simulink model "UAV_Model_LQR"  (R2018a)
settings: Solver=ode45  StartTime=0.0  StopTime=10  RelTol=1e-3  EnableMultiTasking=on
PreLoadFcn:
  | Imported_Data_old
model workspace: external: MAT-File (data not in the file)
values from neighbouring files (symbols this model uses):
  a1 = (Iyy-Izz)/Ixx    (= -0.733333333333)    [Imported_Data.m]
  a2 = Jr/Ixx    (= 0.008)    [Imported_Data.m]
  a3 = (Izz-Ixx)/Iyy    (= 0.733333333333)    [Imported_Data.m]
  a4 = Jr/Iyy    (= 0.008)    [Imported_Data.m]
  a5 = (Ixx-Iyy)/Izz    (= 0)    [Imported_Data.m]
  b1 = l/Ixx    (= 30.6666666667)    [Imported_Data.m]
  b2 = l/Iyy    (= 30.6666666667)    [Imported_Data.m]
  b3 = 1/Izz    (= 76.9230769231)    [Imported_Data.m]
  g = 9.81    [Imported_Data.m]
  K_hover = [5.69569249622213e-13,1.89531365870451e-15,-1.57466857817560e-15,6.95185031132290e-16,8.39284795530529e-14,4.51806830265205e-16,-17.9474107643174,-11.1054776571569,-7.77632326230154e-14,1.88786479489746e-14,2.53644214862947e-13,1.72488798264706e-13;49.1675228808413,10.1590638141113,-1.10370107195727e-12,-7.50360856396961e-15,-3.02757110244610e-14,-5.68697422933292e-16,-1.57487669583132e-15,-3.7779 ...(+585 chars)    [Imported_Data.m]
  K_i = [-9.99999999999991,-5.72733003083861e-14,1.19859349350458e-13;-1.97870657968378e-15,1.52556519389084e-13,7.07106781186449;1.77273448082462e-14,-7.07106781186519,-4.93357134417905e-13;1.93679622698126e-14,-2.41180621006677e-14,-9.68167127074097e-14]    [Imported_Data.m]
  Kf = 3.13e-5    (= 3.13e-05)    [Imported_Data.m]
  KM = 7.5e-7    (= 7.5e-07)    [Imported_Data.m]
  m = 0.650    (= 0.65)    [Imported_Data.m]
  omega_max = (90/100)*9000*(2*pi/(60))    (= 848.230016469)    [Imported_Data.m]
libraries: simulink_extras x3
settings Model: Creator=ahmad  LastModifiedBy=Ahmad
settings DataIOCC: LimitDataPoints=on  SaveFormat=Array
settings OptimizationCC: LifeSpan=inf
settings DebuggingCC: UnderspecifiedInitializationDetection=Classic  MergeDetectMultiDrivingBlocksExec=none  SolverPrmCheckMsg=warning  StateNameClashWarn=warning  SFUnexpectedBacktrackingDiag=warning  SFNoUnconditionalDefaultTransitionDiag=warning  SFExecutionAtInitializationDiag=none
settings HardwareCC: ProdBitPerPointer=32  ProdBitPerSizeT=32  ProdBitPerPtrDiffT=32  ProdLargestAtomicFloat=None  ProdIntDivRoundTo=Undefined  ProdEndianess=Unspecified  ProdWordSize=32  ProdHWDeviceType=32-bit Generic
settings ModelReferenceCC: PropagateSignalLabelsOutOfModel=off
settings CodeAppCC: StateflowObjectComments=on
settings GRTTargetCC: TargetLangStandard=C89/C90 (ANSI)  GeneratePreprocessorConditionals=Disable all
settings ConfigComp: CovMetricSettings=dw  CovHtmlReporting=on  CovSaveCumulativeToWorkspaceVar=on  CovSaveSingleToWorkspaceVar=on  CovExternalEMLEnable=off
settings SimscapeCC: SimscapeNormalizeSystem=off
settings ConfigurationSet: Description=SimMechanics 2G

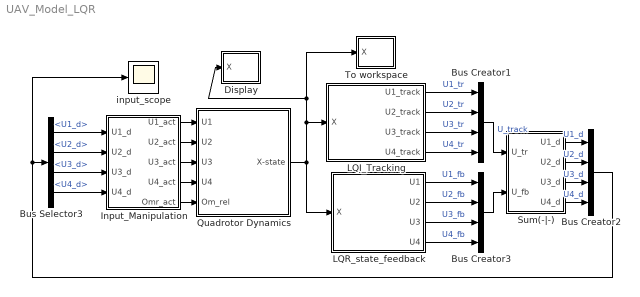
== system UAV_Model_LQR ==
  Bus Creator1 : BusCreator  Inputs=4
  Bus Creator2 : BusCreator  Inputs=4
  Bus Creator3 : BusCreator  Inputs=4
  Bus Selector3 : BusSelector  OutputSignals=U1_d,U2_d,U3_d,U4_d
  Display : Subsystem
  Input_Manipulation : Subsystem
  LQI_Tracking : Subsystem
  LQR_state_feedback : Subsystem
  Quadrotor Dynamics : Subsystem
  Sum(-|-) : Subsystem
  To workspace : Subsystem
  input_scope : Scope
  wires:
  Quadrotor Dynamics/1(X-state) -> LQR_state_feedback/1(X), To workspace/1(X), Display/1(X), LQI_Tracking/1(X)
  LQR_state_feedback/1(U1) -> Bus Creator3/1  "U1_fb"
  LQR_state_feedback/2(U2) -> Bus Creator3/2  "U2_fb"
  LQR_state_feedback/3(U3) -> Bus Creator3/3  "U3_fb"
  LQR_state_feedback/4(U4) -> Bus Creator3/4  "U4_fb"
  Bus Creator3/1 -> Sum(-|-)/2(U_fb)
  Bus Creator2/1 -> input_scope/1, Bus Selector3/1
  Sum(-|-)/1(U1_d) -> Bus Creator2/1  "U1_d"
  Sum(-|-)/2(U2_d) -> Bus Creator2/2  "U2_d"
  Sum(-|-)/3(U3_d) -> Bus Creator2/3  "U3_d"
  Sum(-|-)/4(U4_d) -> Bus Creator2/4  "U4_d"
  LQI_Tracking/1(U1_track) -> Bus Creator1/1  "U1_tr"
  LQI_Tracking/2(U2_track) -> Bus Creator1/2  "U2_tr"
  LQI_Tracking/3(U3_track) -> Bus Creator1/3  "U3_tr"
  Bus Creator1/1 -> Sum(-|-)/1(U_tr)  "U_track"
  LQI_Tracking/4(U4_track) -> Bus Creator1/4  "U4_tr"
  Bus Selector3/1 -> Input_Manipulation/1(U1_d)  "<U1_d>"
  Bus Selector3/2 -> Input_Manipulation/2(U2_d)  "<U2_d>"
  Bus Selector3/3 -> Input_Manipulation/3(U3_d)  "<U3_d>"
  Bus Selector3/4 -> Input_Manipulation/4(U4_d)  "<U4_d>"
  Input_Manipulation/1(U1_act) -> Quadrotor Dynamics/1(U1)
  Input_Manipulation/2(U2_act) -> Quadrotor Dynamics/2(U2)
  Input_Manipulation/3(U3_act) -> Quadrotor Dynamics/3(U3)
  Input_Manipulation/4(U4_act) -> Quadrotor Dynamics/4(U4)
  Input_Manipulation/5(Omr_act) -> Quadrotor Dynamics/5(Om_rel)

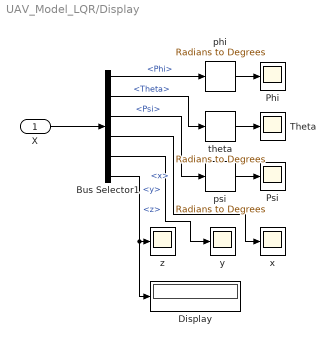
== system UAV_Model_LQR/Display ==
  X : Inport
  Bus Selector1 : BusSelector  OutputSignals=Phi,Theta,Psi,x,y,z
  Display : Display
  Phi : Scope
  Psi : Scope
  "Theta " : Scope
  "phi " : simulink_extras/Transformations/Radians to Degrees
  "psi " : simulink_extras/Transformations/Radians to Degrees
  "theta " : simulink_extras/Transformations/Radians to Degrees
  x : Scope
  y : Scope
  z : Scope
  wires:
  X/1 -> Bus Selector1/1
  Bus Selector1/1 -> "phi "/1  "<Phi>"
  Bus Selector1/2 -> "theta "/1  "<Theta>"
  "theta "/1 -> "Theta "/1
  Bus Selector1/6 -> Display/1, z/1  "<z>"
  Bus Selector1/5 -> y/1  "<y>"
  Bus Selector1/4 -> x/1  "<x>"
  "psi "/1 -> Psi/1
  Bus Selector1/3 -> "psi "/1  "<Psi>"
  "phi "/1 -> Phi/1

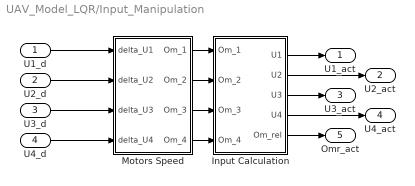
== system UAV_Model_LQR/Input_Manipulation ==
  U1_d : Inport
  U2_d : Inport  Port=2
  U3_d : Inport  Port=3
  U4_d : Inport  Port=4
  Input Calculation : Subsystem
  Motors Speed : Subsystem
  U1_act : Outport
  U2_act : Outport  Port=2
  U3_act : Outport  Port=3
  U4_act : Outport  Port=4
  Omr_act : Outport  Port=5
  wires:
  Input Calculation/1(U1) -> U1_act/1
  Input Calculation/2(U2) -> U2_act/1
  Input Calculation/3(U3) -> U3_act/1
  Input Calculation/4(U4) -> U4_act/1
  Input Calculation/5(Om_rel) -> Omr_act/1
  Motors Speed/1(Om_1) -> Input Calculation/1(Om_1)
  Motors Speed/2(Om_2) -> Input Calculation/2(Om_2)
  Motors Speed/3(Om_3) -> Input Calculation/3(Om_3)
  Motors Speed/4(Om_4) -> Input Calculation/4(Om_4)
  U1_d/1 -> Motors Speed/1(delta_U1)
  U2_d/1 -> Motors Speed/2(delta_U2)
  U3_d/1 -> Motors Speed/3(delta_U3)
  U4_d/1 -> Motors Speed/4(delta_U4)

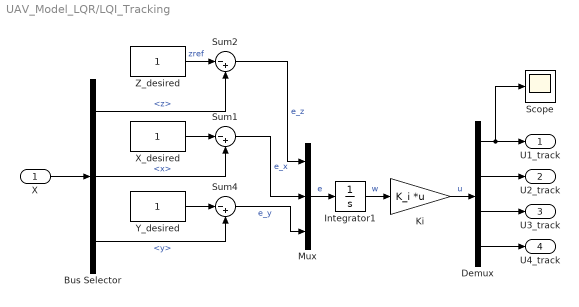
== system UAV_Model_LQR/LQI_Tracking ==
  X : Inport
  Bus Selector : BusSelector  OutputSignals=z,x,y
  Demux : Demux
  Integrator1 : Integrator
  Ki : Gain  Gain=K_i  Multiplication=Matrix(K*u)
  Mux : Mux  Inputs=3
  Scope : Scope
  Sum1 : Sum  Inputs=|-+
  Sum2 : Sum  Inputs=|-+
  Sum4 : Sum  Inputs=|-+
  X_desired : Constant
  Y_desired : Constant
  Z_desired : Constant
  U1_track : Outport
  U2_track : Outport  Port=2
  U3_track : Outport  Port=3
  U4_track : Outport  Port=4
  wires:
  X/1 -> Bus Selector/1
  Demux/1 -> Scope/1, U1_track/1
  Demux/2 -> U2_track/1
  Demux/3 -> U3_track/1
  Demux/4 -> U4_track/1
  Z_desired/1 -> Sum2/1  "zref"
  Ki/1 -> Demux/1  "u"
  Bus Selector/1 -> Sum2/2  "<z>"
  X_desired/1 -> Sum1/1
  Y_desired/1 -> Sum4/1
  Sum1/1 -> Mux/2  "e_x"
  Sum4/1 -> Mux/3  "e_y"
  Sum2/1 -> Mux/1  "e_z"
  Mux/1 -> Integrator1/1  "e"
  Integrator1/1 -> Ki/1  "w"
  Bus Selector/2 -> Sum1/2  "<x>"
  Bus Selector/3 -> Sum4/2  "<y>"

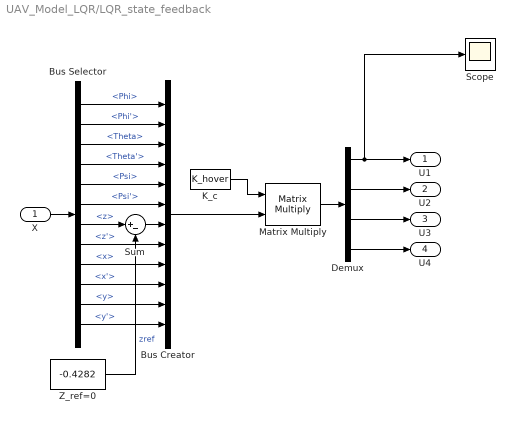
== system UAV_Model_LQR/LQR_state_feedback ==
  X : Inport
  Bus Creator : BusCreator  Inputs=12
  Bus Selector : BusSelector  OutputSignals=Phi,Phi',Theta,Theta',Psi,Psi',z,z',x,x',y,y'
  Demux : Demux
  K_c : Constant  Value=K_hover
  Matrix Multiply : Product  Multiplication=Matrix(*)
  Scope : Scope
  Sum : Sum  Inputs=|+-
  Z_ref=0 : Constant  Value=-0.4282
  U1 : Outport
  U2 : Outport  Port=2
  U3 : Outport  Port=3
  U4 : Outport  Port=4
  wires:
  X/1 -> Bus Selector/1
  Bus Selector/1 -> Bus Creator/1  "<Phi>"
  Bus Selector/2 -> Bus Creator/2  "<Phi'>"
  Bus Selector/3 -> Bus Creator/3  "<Theta>"
  Bus Selector/4 -> Bus Creator/4  "<Theta'>"
  Bus Creator/1 -> Matrix Multiply/2
  K_c/1 -> Matrix Multiply/1
  Bus Selector/7 -> Sum/1  "<z>"
  Bus Selector/8 -> Bus Creator/8  "<z'>"
  Bus Selector/9 -> Bus Creator/9  "<x>"
  Bus Selector/10 -> Bus Creator/10  "<x'>"
  Bus Selector/11 -> Bus Creator/11  "<y>"
  Bus Selector/12 -> Bus Creator/12  "<y'>"
  Z_ref=0/1 -> Sum/2  "zref"
  Sum/1 -> Bus Creator/7
  Demux/1 -> U1/1, Scope/1
  Matrix Multiply/1 -> Demux/1
  Bus Selector/5 -> Bus Creator/5  "<Psi>"
  Bus Selector/6 -> Bus Creator/6  "<Psi'>"
  Demux/2 -> U2/1
  Demux/3 -> U3/1
  Demux/4 -> U4/1

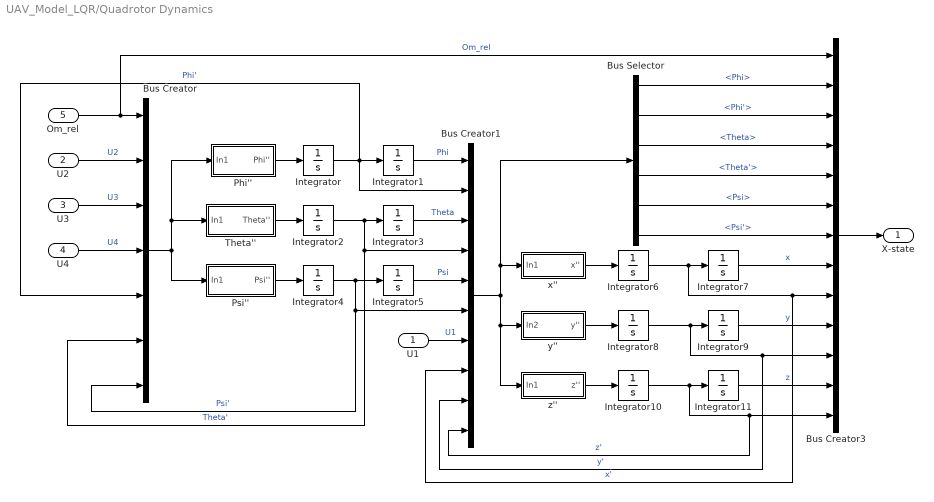
== system UAV_Model_LQR/Quadrotor Dynamics ==
  U1 : Inport
  U2 : Inport  Port=2
  U3 : Inport  Port=3
  U4 : Inport  Port=4
  Om_rel : Inport  Port=5
  Bus Creator : BusCreator  Inputs=7
  Bus Creator1 : BusCreator  Inputs=10
  Bus Creator3 : BusCreator  Inputs=13
  Bus Selector : BusSelector  OutputSignals=Phi,Phi',Theta,Theta',Psi,Psi'
  Integrator{,1..11} (12 alike) : Integrator
  Phi'' : Subsystem
  Psi'' : Subsystem
  Theta'' : Subsystem
  x'' : Subsystem
  y'' : Subsystem
  z'' : Subsystem
  X-state : Outport
  wires:
  Bus Creator/1 -> Phi''/1(In1), Theta''/1(In1), Psi''/1(In1)
  Theta''/1(Theta'') -> Integrator2/1
  Phi''/1(Phi'') -> Integrator/1
  Psi''/1(Psi'') -> Integrator4/1
  Integrator4/1 -> Bus Creator/7, Bus Creator1/6, Integrator5/1  "Psi'"
  Integrator2/1 -> Bus Creator/6, Bus Creator1/4, Integrator3/1  "Theta'"
  Integrator/1 -> Bus Creator1/2, Integrator1/1, Bus Creator/5  "Phi'"
  Om_rel/1 -> Bus Creator3/1, Bus Creator/1  "Om_rel"
  U2/1 -> Bus Creator/2  "U2"
  U3/1 -> Bus Creator/3  "U3"
  U4/1 -> Bus Creator/4  "U4"
  Integrator1/1 -> Bus Creator1/1  "Phi"
  Integrator3/1 -> Bus Creator1/3  "Theta"
  Integrator5/1 -> Bus Creator1/5  "Psi"
  x''/1(x'') -> Integrator6/1
  Integrator6/1 -> Bus Creator3/9, Bus Creator1/8, Integrator7/1  "x'"
  Integrator8/1 -> Integrator9/1, Bus Creator3/11, Bus Creator1/9  "y'"
  Integrator10/1 -> Integrator11/1, Bus Creator3/13, Bus Creator1/10  "z'"
  y''/1(y'') -> Integrator8/1
  z''/1(z'') -> Integrator10/1
  Bus Selector/1 -> Bus Creator3/2  "<Phi>"
  Bus Selector/2 -> Bus Creator3/3  "<Phi'>"
  Bus Selector/3 -> Bus Creator3/4  "<Theta>"
  Bus Selector/4 -> Bus Creator3/5  "<Theta'>"
  Bus Selector/5 -> Bus Creator3/6  "<Psi>"
  Bus Selector/6 -> Bus Creator3/7  "<Psi'>"
  Bus Creator1/1 -> z''/1(In1), y''/1(In2), Bus Selector/1, x''/1(In1)
  Integrator7/1 -> Bus Creator3/8  "x"
  Integrator9/1 -> Bus Creator3/10  "y"
  Integrator11/1 -> Bus Creator3/12  "z"
  U1/1 -> Bus Creator1/7  "U1"
  Bus Creator3/1 -> X-state/1

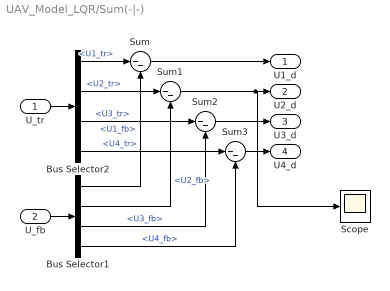
== system UAV_Model_LQR/Sum(-|-) ==
  U_tr : Inport
  U_fb : Inport  Port=2
  Bus Selector1 : BusSelector  OutputSignals=U1_fb,U2_fb,U3_fb,U4_fb
  Bus Selector2 : BusSelector  OutputSignals=U1_tr,U2_tr,U3_tr,U4_tr
  Scope : Scope
  Sum{,1..3} (4 alike) : Sum  Inputs=|--
  U1_d : Outport
  U2_d : Outport  Port=2
  U3_d : Outport  Port=3
  U4_d : Outport  Port=4
  wires:
  U_fb/1 -> Bus Selector1/1
  Bus Selector1/1 -> Sum/2  "<U1_fb>"
  Bus Selector1/2 -> Sum1/2  "<U2_fb>"
  Bus Selector1/3 -> Sum2/2  "<U3_fb>"
  Bus Selector1/4 -> Sum3/2  "<U4_fb>"
  Sum/1 -> U1_d/1
  Sum1/1 -> Scope/1, U2_d/1
  Sum2/1 -> U3_d/1
  Sum3/1 -> U4_d/1
  Bus Selector2/3 -> Sum2/1  "<U3_tr>"
  U_tr/1 -> Bus Selector2/1
  Bus Selector2/1 -> Sum/1  "<U1_tr>"
  Bus Selector2/2 -> Sum1/1  "<U2_tr>"
  Bus Selector2/4 -> Sum3/1  "<U4_tr>"

== system UAV_Model_LQR/To workspace ==
  X : Inport
  Bus Selector2 : BusSelector  OutputSignals=Phi,Theta,Psi,z,y,x
  phi_out : ToWorkspace  VariableName=Phi_out  SaveFormat=Timeseries  SampleTime=-1
  psi_out : ToWorkspace  VariableName=Psi_out  SaveFormat=Timeseries  SampleTime=-1
  theta_out : ToWorkspace  VariableName=Theta_out  SaveFormat=Timeseries  SampleTime=-1
  x_out : ToWorkspace  VariableName=x_out  SaveFormat=Timeseries  SampleTime=-1
  y_out : ToWorkspace  VariableName=y_out  SaveFormat=Timeseries  SampleTime=-1
  z_out : ToWorkspace  VariableName=z_out  SaveFormat=Timeseries  SampleTime=-1
  wires:
  Bus Selector2/1 -> phi_out/1  "<Phi>"
  Bus Selector2/2 -> theta_out/1  "<Theta>"
  Bus Selector2/3 -> psi_out/1  "<Psi>"
  Bus Selector2/4 -> z_out/1  "<z>"
  X/1 -> Bus Selector2/1
  Bus Selector2/5 -> y_out/1  "<y>"
  Bus Selector2/6 -> x_out/1  "<x>"

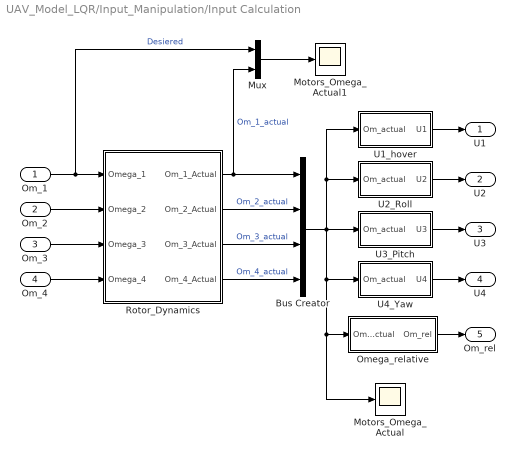
== system UAV_Model_LQR/Input_Manipulation/Input Calculation ==
  Om_1 : Inport
  Om_2 : Inport  Port=2
  Om_3 : Inport  Port=3
  Om_4 : Inport  Port=4
  Bus Creator : BusCreator  Inputs=4
  Motors_Omega_Actual : Scope
  Motors_Omega_Actual1 : Scope
  Mux : Mux  Inputs=2
  Omega_relative : Subsystem
  Rotor_Dynamics : Subsystem
  U1_hover : Subsystem
  U2_Roll : Subsystem
  U3_Pitch : Subsystem
  U4_Yaw : Subsystem
  U1 : Outport
  U2 : Outport  Port=2
  U3 : Outport  Port=3
  U4 : Outport  Port=4
  Om_rel : Outport  Port=5
  wires:
  Om_1/1 -> Mux/1, Rotor_Dynamics/1(Omega_1)  "Desiered"
  Om_3/1 -> Rotor_Dynamics/3(Omega_3)
  Om_2/1 -> Rotor_Dynamics/2(Omega_2)
  Om_4/1 -> Rotor_Dynamics/4(Omega_4)
  Rotor_Dynamics/1(Om_1_Actual) -> Mux/2, Bus Creator/1  "Om_1_actual"
  Rotor_Dynamics/2(Om_2_Actual) -> Bus Creator/2  "Om_2_actual"
  Rotor_Dynamics/3(Om_3_Actual) -> Bus Creator/3  "Om_3_actual"
  Rotor_Dynamics/4(Om_4_Actual) -> Bus Creator/4  "Om_4_actual"
  Bus Creator/1 -> U3_Pitch/1(Om_actual), U4_Yaw/1(Om_actual), Omega_relative/1(Om_actual), Motors_Omega_Actual/1, U2_Roll/1(Om_actual), U1_hover/1(Om_actual)
  U1_hover/1(U1) -> U1/1
  U2_Roll/1(U2) -> U2/1
  U3_Pitch/1(U3) -> U3/1
  U4_Yaw/1(U4) -> U4/1
  Omega_relative/1(Om_rel) -> Om_rel/1
  Mux/1 -> Motors_Omega_Actual1/1

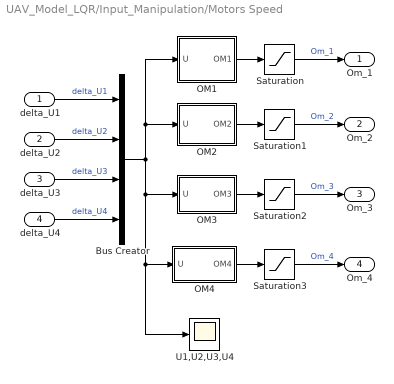
== system UAV_Model_LQR/Input_Manipulation/Motors Speed ==
  delta_U1 : Inport
  delta_U2 : Inport  Port=2
  delta_U3 : Inport  Port=3
  delta_U4 : Inport  Port=4
  Bus Creator : BusCreator  Inputs=4
  OM1 : Subsystem
  OM2 : Subsystem
  OM3 : Subsystem
  OM4 : Subsystem
  Saturation{,1..3} (4 alike) : Saturate  UpperLimit=omega_max  LowerLimit=0
  U1,U2,U3,U4 : Scope
  Om_1 : Outport
  Om_2 : Outport  Port=2
  Om_3 : Outport  Port=3
  Om_4 : Outport  Port=4
  wires:
  delta_U1/1 -> Bus Creator/1  "delta_U1"
  delta_U4/1 -> Bus Creator/4  "delta_U4"
  delta_U3/1 -> Bus Creator/3  "delta_U3"
  delta_U2/1 -> Bus Creator/2  "delta_U2"
  Bus Creator/1 -> OM1/1(U), OM2/1(U), U1,U2,U3,U4/1, OM4/1(U), OM3/1(U)
  OM1/1(OM1) -> Saturation/1
  OM2/1(OM2) -> Saturation1/1
  OM3/1(OM3) -> Saturation2/1
  OM4/1(OM4) -> Saturation3/1
  Saturation3/1 -> Om_4/1  "Om_4"
  Saturation2/1 -> Om_3/1  "Om_3"
  Saturation1/1 -> Om_2/1  "Om_2"
  Saturation/1 -> Om_1/1  "Om_1"

== system UAV_Model_LQR/Quadrotor Dynamics/Phi'' ==
  In1 : Inport
  Bus Selector : BusSelector  OutputSignals=Psi',Theta',Om_rel,U2
  Mux : Mux  Inputs=7
  Phi_dot_dot : Fcn  Expr=u(1)*u(2)*u(3)-u(3)*u(4)*u(5)+u(6)*u(7)
  a1 : Constant  Value=a1
  a2 : Constant  Value=a2
  b1 : Constant  Value=b1
  Phi'' : Outport
  wires:
  In1/1 -> Bus Selector/1
  a1/1 -> Mux/2
  Bus Selector/1 -> Mux/1  "<Psi'>"
  Bus Selector/2 -> Mux/3  "<Theta'>"
  Bus Selector/3 -> Mux/4  "<Om_rel>"
  a2/1 -> Mux/5
  Bus Selector/4 -> Mux/6  "<U2>"
  b1/1 -> Mux/7
  Mux/1 -> Phi_dot_dot/1
  Phi_dot_dot/1 -> Phi''/1

== system UAV_Model_LQR/Quadrotor Dynamics/Psi'' ==
  In1 : Inport
  Add : Sum
  Bus Selector : BusSelector  OutputSignals=Phi',Theta',U4
  Product1 : Product  Inputs=3
  Product2 : Product
  a5 : Constant  Value=a5
  b3 : Constant  Value=b3
  Psi'' : Outport
  wires:
  In1/1 -> Bus Selector/1
  b3/1 -> Product2/2
  a5/1 -> Product1/1
  Add/1 -> Psi''/1
  Bus Selector/1 -> Product1/2  "<Phi'>"
  Bus Selector/2 -> Product1/3  "<Theta'>"
  Bus Selector/3 -> Product2/1  "<U4>"
  Product2/1 -> Add/2
  Product1/1 -> Add/1

== system UAV_Model_LQR/Quadrotor Dynamics/Theta'' ==
  In1 : Inport
  Add : Sum  Inputs=+++
  Bus Selector : BusSelector  OutputSignals=Psi',Phi',Om_rel,U3
  Product1 : Product  Inputs=3
  Product2 : Product  Inputs=3
  Product3 : Product
  a3 : Constant  Value=a3
  a4 : Constant  Value=a4
  b2 : Constant  Value=b2
  Theta'' : Outport
  wires:
  b2/1 -> Product3/2
  a3/1 -> Product1/1
  Product3/1 -> Add/3
  Product1/1 -> Add/2
  Product2/1 -> Add/1
  Add/1 -> Theta''/1
  Bus Selector/4 -> Product3/1  "<U3>"
  Bus Selector/1 -> Product1/2  "<Psi'>"
  Bus Selector/2 -> Product2/1, Product1/3  "<Phi'>"
  Bus Selector/3 -> Product2/2  "<Om_rel>"
  a4/1 -> Product2/3
  In1/1 -> Bus Selector/1

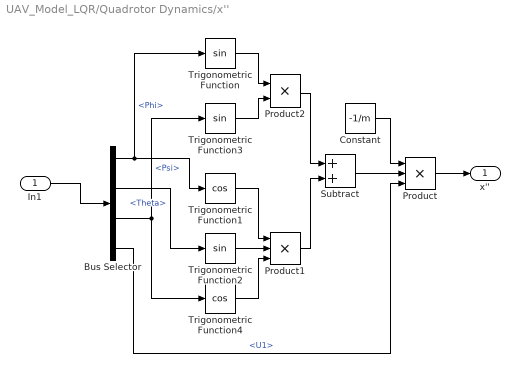
== system UAV_Model_LQR/Quadrotor Dynamics/x'' ==
  In1 : Inport
  Bus Selector : BusSelector  OutputSignals=Phi,Theta,Psi,U1
  Constant : Constant  Value=-1/m
  Product : Product  Inputs=3
  Product1 : Product  Inputs=3
  Product2 : Product
  Subtract : Sum
  Trigonometric Function : Trigonometry
  Trigonometric Function1 : Trigonometry  Operator=cos
  Trigonometric Function2 : Trigonometry
  Trigonometric Function3 : Trigonometry
  Trigonometric Function4 : Trigonometry  Operator=cos
  x'' : Outport
  wires:
  In1/1 -> Bus Selector/1
  Bus Selector/1 -> Trigonometric Function1/1, Trigonometric Function/1  "<Phi>"
  Bus Selector/3 -> Trigonometric Function3/1, Trigonometric Function4/1  "<Psi>"
  Trigonometric Function/1 -> Product2/1
  Trigonometric Function3/1 -> Product2/2
  Bus Selector/2 -> Trigonometric Function2/1  "<Theta>"
  Trigonometric Function2/1 -> Product1/2
  Trigonometric Function1/1 -> Product1/1
  Trigonometric Function4/1 -> Product1/3
  Product2/1 -> Subtract/1
  Product1/1 -> Subtract/2
  Bus Selector/4 -> Product/3  "<U1>"
  Subtract/1 -> Product/2
  Constant/1 -> Product/1
  Product/1 -> x''/1

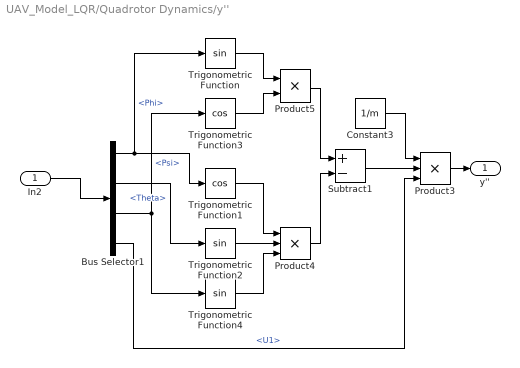
== system UAV_Model_LQR/Quadrotor Dynamics/y'' ==
  In2 : Inport
  Bus Selector1 : BusSelector  OutputSignals=Phi,Theta,Psi,U1
  Constant3 : Constant  Value=1/m
  Product3 : Product  Inputs=3
  Product4 : Product  Inputs=3
  Product5 : Product
  Subtract1 : Sum  Inputs=+-
  Trigonometric Function : Trigonometry
  Trigonometric Function1 : Trigonometry  Operator=cos
  Trigonometric Function2 : Trigonometry
  Trigonometric Function3 : Trigonometry  Operator=cos
  Trigonometric Function4 : Trigonometry
  y'' : Outport
  wires:
  In2/1 -> Bus Selector1/1
  Bus Selector1/1 -> Trigonometric Function1/1, Trigonometric Function/1  "<Phi>"
  Bus Selector1/3 -> Trigonometric Function3/1, Trigonometric Function4/1  "<Psi>"
  Trigonometric Function/1 -> Product5/1
  Trigonometric Function3/1 -> Product5/2
  Bus Selector1/2 -> Trigonometric Function2/1  "<Theta>"
  Trigonometric Function2/1 -> Product4/2
  Trigonometric Function1/1 -> Product4/1
  Trigonometric Function4/1 -> Product4/3
  Product5/1 -> Subtract1/1
  Product4/1 -> Subtract1/2
  Bus Selector1/4 -> Product3/3  "<U1>"
  Subtract1/1 -> Product3/2
  Constant3/1 -> Product3/1
  Product3/1 -> y''/1

== system UAV_Model_LQR/Quadrotor Dynamics/z'' ==
  In1 : Inport
  Bus Selector : BusSelector  OutputSignals=Phi,Theta,U1
  Constant : Constant  Value=1/m
  Constant1 : Constant  Value=g
  Product : Product  Inputs=3
  Product2 : Product
  Subtract : Sum  Inputs=-+
  Trigonometric Function : Trigonometry  Operator=cos
  Trigonometric Function3 : Trigonometry  Operator=cos
  z'' : Outport
  wires:
  In1/1 -> Bus Selector/1
  Trigonometric Function/1 -> Product2/1
  Trigonometric Function3/1 -> Product2/2
  Bus Selector/1 -> Trigonometric Function/1  "<Phi>"
  Bus Selector/2 -> Trigonometric Function3/1  "<Theta>"
  Product2/1 -> Product/2
  Bus Selector/3 -> Product/3  "<U1>"
  Constant/1 -> Product/1
  Constant1/1 -> Subtract/2
  Product/1 -> Subtract/1
  Subtract/1 -> z''/1

== system UAV_Model_LQR/Input_Manipulation/Input Calculation/Omega_relative ==
  Om_actual : Inport
  Add : Sum  Inputs=-+-+
  Bus Selector : BusSelector  OutputSignals=Om_1_actual,Om_2_actual,Om_3_actual,Om_4_actual
  Om_rel : Outport
  wires:
  Om_actual/1 -> Bus Selector/1
  Bus Selector/1 -> Add/1  "<Om_1_actual>"
  Bus Selector/2 -> Add/2  "<Om_2_actual>"
  Bus Selector/3 -> Add/3  "<Om_3_actual>"
  Bus Selector/4 -> Add/4  "<Om_4_actual>"
  Add/1 -> Om_rel/1

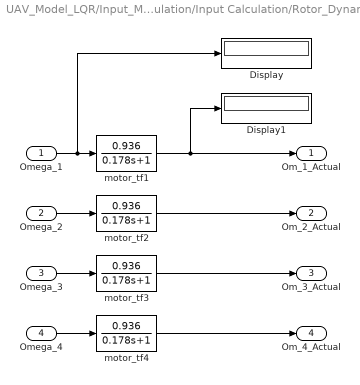
== system UAV_Model_LQR/Input_Manipulation/Input Calculation/Rotor_Dynamics ==
  Omega_1 : Inport
  Omega_2 : Inport  Port=2
  Omega_3 : Inport  Port=3
  Omega_4 : Inport  Port=4
  Display : Display
  Display1 : Display
  motor_tf{1..4} (4 alike) : TransferFcn  Numerator=[0.936]  Denominator=[0.178 1]
  Om_1_Actual : Outport
  Om_2_Actual : Outport  Port=2
  Om_3_Actual : Outport  Port=3
  Om_4_Actual : Outport  Port=4
  wires:
  motor_tf2/1 -> Om_2_Actual/1
  motor_tf3/1 -> Om_3_Actual/1
  motor_tf1/1 -> Display1/1, Om_1_Actual/1
  motor_tf4/1 -> Om_4_Actual/1
  Omega_1/1 -> Display/1, motor_tf1/1
  Omega_2/1 -> motor_tf2/1
  Omega_3/1 -> motor_tf3/1
  Omega_4/1 -> motor_tf4/1

== system UAV_Model_LQR/Input_Manipulation/Input Calculation/U1_hover ==
  Om_actual : Inport
  Add : Sum  Inputs=++++
  Bus Selector : BusSelector  OutputSignals=Om_1_actual,Om_2_actual,Om_3_actual,Om_4_actual
  Math Function{,1..3} (4 alike) : Math  Operator=square  SaturateOnIntegerOverflow=on
  Product : Product
  Thrust Coefficient : Constant  Value=Kf
  U1 : Outport
  wires:
  Om_actual/1 -> Bus Selector/1
  Thrust Coefficient/1 -> Product/1
  Add/1 -> Product/2
  Math Function/1 -> Add/1
  Math Function3/1 -> Add/2
  Math Function2/1 -> Add/3
  Math Function1/1 -> Add/4
  Bus Selector/1 -> Math Function/1  "<Om_1_actual>"
  Bus Selector/2 -> Math Function3/1  "<Om_2_actual>"
  Bus Selector/3 -> Math Function2/1  "<Om_3_actual>"
  Bus Selector/4 -> Math Function1/1  "<Om_4_actual>"
  Product/1 -> U1/1

== system UAV_Model_LQR/Input_Manipulation/Input Calculation/U2_Roll ==
  Om_actual : Inport
  Add : Sum  Inputs=-+
  Bus Selector : BusSelector  OutputSignals=Om_2_actual,Om_4_actual
  Om2^2 : Math  Operator=square  SaturateOnIntegerOverflow=on
  Om4^2 : Math  Operator=square  SaturateOnIntegerOverflow=on
  Product : Product
  Thrust Coefficient : Constant  Value=Kf
  U2 : Outport
  wires:
  Thrust Coefficient/1 -> Product/1
  Add/1 -> Product/2
  Om2^2/1 -> Add/1
  Om4^2/1 -> Add/2
  Bus Selector/1 -> Om2^2/1  "<Om_2_actual>"
  Bus Selector/2 -> Om4^2/1  "<Om_4_actual>"
  Product/1 -> U2/1
  Om_actual/1 -> Bus Selector/1

== system UAV_Model_LQR/Input_Manipulation/Input Calculation/U3_Pitch ==
  Om_actual : Inport
  Add : Sum  Inputs=+-
  Bus Selector : BusSelector  OutputSignals=Om_1_actual,Om_3_actual
  Om1^2 : Math  Operator=square  SaturateOnIntegerOverflow=on
  Om3^2 : Math  Operator=square  SaturateOnIntegerOverflow=on
  Product : Product
  Thrust Coefficient : Constant  Value=Kf
  U3 : Outport
  wires:
  Thrust Coefficient/1 -> Product/1
  Add/1 -> Product/2
  Om1^2/1 -> Add/1
  Om3^2/1 -> Add/2
  Product/1 -> U3/1
  Om_actual/1 -> Bus Selector/1
  Bus Selector/1 -> Om1^2/1  "<Om_1_actual>"
  Bus Selector/2 -> Om3^2/1  "<Om_3_actual>"

== system UAV_Model_LQR/Input_Manipulation/Input Calculation/U4_Yaw ==
  Om_actual : Inport
  Add : Sum  Inputs=+-+-
  Bus Selector : BusSelector  OutputSignals=Om_1_actual,Om_2_actual,Om_3_actual,Om_4_actual
  Math Function{,1..3} (4 alike) : Math  Operator=square  SaturateOnIntegerOverflow=on
  Moment Coefficient : Constant  Value=KM
  Product : Product
  U4 : Outport
  wires:
  Om_actual/1 -> Bus Selector/1
  Moment Coefficient/1 -> Product/1
  Add/1 -> Product/2
  Math Function/1 -> Add/1
  Math Function3/1 -> Add/2
  Math Function2/1 -> Add/3
  Math Function1/1 -> Add/4
  Bus Selector/1 -> Math Function/1  "<Om_1_actual>"
  Bus Selector/2 -> Math Function3/1  "<Om_2_actual>"
  Bus Selector/3 -> Math Function2/1  "<Om_3_actual>"
  Bus Selector/4 -> Math Function1/1  "<Om_4_actual>"
  Product/1 -> U4/1

== system UAV_Model_LQR/Input_Manipulation/Motors Speed/OM1 ==
  U : Inport
  Bus Selector : BusSelector  OutputSignals=delta_U1,delta_U3,delta_U4
  Constant : Constant  Value=1/(4*Kf)
  Constant1 : Constant  Value=1/(2*Kf)
  Constant2 : Constant  Value=1/(4*KM)
  Product : Product
  Product1 : Product
  Product2 : Product
  Sqrt : Sqrt  SaturateOnIntegerOverflow=on
  Subtract : Sum  Inputs=+++
  OM1 : Outport
  wires:
  U/1 -> Bus Selector/1
  Bus Selector/2 -> Product1/1  "<delta_U3>"
  Bus Selector/1 -> Product/1  "<delta_U1>"
  Bus Selector/3 -> Product2/1  "<delta_U4>"
  Product/1 -> Subtract/1
  Product1/1 -> Subtract/2
  Product2/1 -> Subtract/3
  Constant1/1 -> Product1/2
  Constant/1 -> Product/2
  Constant2/1 -> Product2/2
  Subtract/1 -> Sqrt/1
  Sqrt/1 -> OM1/1

== system UAV_Model_LQR/Input_Manipulation/Motors Speed/OM2 ==
  U : Inport
  Bus Selector : BusSelector  OutputSignals=delta_U1,delta_U2,delta_U4
  Constant : Constant  Value=1/(4*Kf)
  Constant1 : Constant  Value=1/(2*Kf)
  Constant2 : Constant  Value=1/(4*KM)
  Product : Product
  Product1 : Product
  Product2 : Product
  Sqrt : Sqrt  SaturateOnIntegerOverflow=on
  Subtract : Sum  Inputs=+--
  OM2 : Outport
  wires:
  U/1 -> Bus Selector/1
  Bus Selector/2 -> Product1/1  "<delta_U2>"
  Bus Selector/1 -> Product/1  "<delta_U1>"
  Bus Selector/3 -> Product2/1  "<delta_U4>"
  Product/1 -> Subtract/1
  Product1/1 -> Subtract/2
  Product2/1 -> Subtract/3
  Subtract/1 -> Sqrt/1
  Constant1/1 -> Product1/2
  Constant/1 -> Product/2
  Constant2/1 -> Product2/2
  Sqrt/1 -> OM2/1

== system UAV_Model_LQR/Input_Manipulation/Motors Speed/OM3 ==
  U : Inport
  Bus Selector : BusSelector  OutputSignals=delta_U1,delta_U3,delta_U4
  Constant : Constant  Value=1/(4*Kf)
  Constant1 : Constant  Value=1/(2*Kf)
  Constant2 : Constant  Value=1/(4*KM)
  Product : Product
  Product1 : Product
  Product2 : Product
  Sqrt : Sqrt  SaturateOnIntegerOverflow=on
  Subtract : Sum  Inputs=+-+
  OM3 : Outport
  wires:
  U/1 -> Bus Selector/1
  Bus Selector/2 -> Product1/1  "<delta_U3>"
  Bus Selector/1 -> Product/1  "<delta_U1>"
  Bus Selector/3 -> Product2/1  "<delta_U4>"
  Product/1 -> Subtract/1
  Product1/1 -> Subtract/2
  Product2/1 -> Subtract/3
  Subtract/1 -> Sqrt/1
  Constant1/1 -> Product1/2
  Constant/1 -> Product/2
  Constant2/1 -> Product2/2
  Sqrt/1 -> OM3/1

== system UAV_Model_LQR/Input_Manipulation/Motors Speed/OM4 ==
  U : Inport
  Bus Selector : BusSelector  OutputSignals=delta_U1,delta_U2,delta_U4
  Constant : Constant  Value=1/(4*Kf)
  Constant1 : Constant  Value=1/(2*Kf)
  Constant2 : Constant  Value=1/(4*KM)
  Product : Product
  Product1 : Product
  Product2 : Product
  Sqrt : Sqrt  SaturateOnIntegerOverflow=on
  Subtract : Sum  Inputs=++-
  OM4 : Outport
  wires:
  U/1 -> Bus Selector/1
  Bus Selector/2 -> Product1/1  "<delta_U2>"
  Bus Selector/1 -> Product/1  "<delta_U1>"
  Bus Selector/3 -> Product2/1  "<delta_U4>"
  Product/1 -> Subtract/1
  Product1/1 -> Subtract/2
  Product2/1 -> Subtract/3
  Subtract/1 -> Sqrt/1
  Constant1/1 -> Product1/2
  Constant/1 -> Product/2
  Constant2/1 -> Product2/2
  Sqrt/1 -> OM4/1
